simulink model "Lcontainer_sim"  (R2018b)
settings: Solver=ode1  StartTime=0.0  StopTime=600  FixedStep=0.1  RelTol=1e-3
libraries: neural x49, simulink x2
(part 2 of 2)

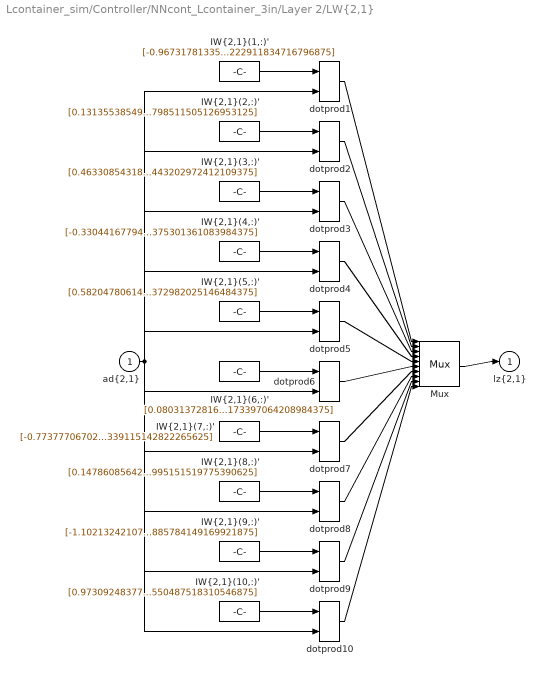
== system Lcontainer_sim/Controller/NNcont_Lcontainer_3in/Layer 2/LW{2,1} ==
  "ad{2,1}" : Inport  PortDimensions=10
      mask Display: e = 0.06;c1 = [120 230 180]/255;c2 = ([120 230 180]+0)/(256+128);c3 = ([120 230 180]+128)/(256+128);patch([0 1 1 0],[0 0 1 1],c1);patch([0 1 1 1-e 1-e 0+e],[0 0 1 1-e 0+e 0+e],c2);patch([0 0 1 1-e 0+e 0+e],[0 1 1 1-e 1-e 0+e],c3);plot([0 1 1 0 0],[0 0 1 1 0]);
  "IW{2,1}(1,:)'" : Constant  Value=[-0.9673178133559503510952026772429235279560089111328125;0.53839778171147634200366383083746768534183502197265625;-0.722317642025362971480717533268034458160400390625;0.8553552777126747219682556533371098339557647705078125;0.275878338813815293661946270731277763843536376953125;-0.02755546810020788328632335151269217021763324737548828125;0.82237984032601907369297578043187968432903289794921875;-0.2547472202517508943486745920381508767604827880859375;-0.61557536337765605960470338686718605458736419677734375;0.153664159931131638625600999148446135222911834716796875]
      mask Display: e = 0.06;c1 = [120 150 230]/255;c2 = ([120 150 230]+0)/383;c3 = ([120 150 230]+128)/383;patch([0 1 1 0],[0 0 1 1],c1);patch([0 1 1 1-e 1-e 0+e],[0 0 1 1-e 0+e 0+e],c2);patch([0 0 1 1-e 0+e 0+e],[0 1 1 1-e 1-e 0+e],c3);plot([0 1 1 0 0],[0 0 1 1 0]);disp('weights');
  "IW{2,1}(10,:)'" : Constant  Value=[0.97309248377746315750158601076691411435604095458984375;-0.845856659992735959718856975086964666843414306640625;0.0295346903368784718946216116819414310157299041748046875;-1.1110911960074727478087197596323676407337188720703125;0.3060928624502607942048371114651672542095184326171875;-0.026387217399169611564690995919590932317078113555908203125;-0.554579983764879269614311851910315454006195068359375;-0.7959887047101454893294203429832123219966888427734375;-0.53675247865637409905303911727969534695148468017578125;-0.30786197281541471948429489202680997550487518310546875]
      mask Display: e = 0.06;c1 = [120 150 230]/255;c2 = ([120 150 230]+0)/383;c3 = ([120 150 230]+128)/383;patch([0 1 1 0],[0 0 1 1],c1);patch([0 1 1 1-e 1-e 0+e],[0 0 1 1-e 0+e 0+e],c2);patch([0 0 1 1-e 0+e 0+e],[0 1 1 1-e 1-e 0+e],c3);plot([0 1 1 0 0],[0 0 1 1 0]);disp('weights');
  "IW{2,1}(2,:)'" : Constant  Value=[0.1313553854999522096935749004842364229261875152587890625;-0.79774829886561471337103057521744631230831146240234375;-0.286014502405725845601835999332251958549022674560546875;1.1879656245342637976847299796645529568195343017578125;-0.70701622775883998794910212382092140614986419677734375;0.1677083387146580395477002412008005194365978240966796875;-0.46969451886407587171134991876897402107715606689453125;-0.138127570352924611274403332572546787559986114501953125;-0.43525645097113885295669888364500366151332855224609375;0.050289888408718404211317221097488072700798511505126953125]
      mask Display: e = 0.06;c1 = [120 150 230]/255;c2 = ([120 150 230]+0)/383;c3 = ([120 150 230]+128)/383;patch([0 1 1 0],[0 0 1 1],c1);patch([0 1 1 1-e 1-e 0+e],[0 0 1 1-e 0+e 0+e],c2);patch([0 0 1 1-e 0+e 0+e],[0 1 1 1-e 1-e 0+e],c3);plot([0 1 1 0 0],[0 0 1 1 0]);disp('weights');
  "IW{2,1}(3,:)'" : Constant  Value=[0.463308543185886156923203316182480193674564361572265625;0.01474050328529204374750083417211499181576073169708251953125;0.5708458173938455448848117157467640936374664306640625;-0.36304390338556735695618726822431199252605438232421875;0.03802927902901009904468310196534730494022369384765625;0.8688905579410917123794888539123348891735076904296875;-0.368022670402931073585506283052382059395313262939453125;1.078571025995817223019912489689886569976806640625;-0.42042514591632340614779650422860868275165557861328125;0.449357619793621321235832510865293443202972412109375]
      mask Display: e = 0.06;c1 = [120 150 230]/255;c2 = ([120 150 230]+0)/383;c3 = ([120 150 230]+128)/383;patch([0 1 1 0],[0 0 1 1],c1);patch([0 1 1 1-e 1-e 0+e],[0 0 1 1-e 0+e 0+e],c2);patch([0 0 1 1-e 0+e 0+e],[0 1 1 1-e 1-e 0+e],c3);plot([0 1 1 0 0],[0 0 1 1 0]);disp('weights');
  "IW{2,1}(4,:)'" : Constant  Value=[-0.330441677946859357906106424707104451954364776611328125;0.9398932320279040908417300670407712459564208984375;0.024098708014007048927584975217541796155273914337158203125;0.4618698985408240531569390441291034221649169921875;-1.1397682984094237301775365267531014978885650634765625;0.860210379926586110599373569129966199398040771484375;-0.17513721026530471025495216963463462889194488525390625;-0.410569653732319128636163441115058958530426025390625;-0.5560344839229272029257344911457039415836334228515625;-0.308418252656767977182283857473521493375301361083984375]
      mask Display: e = 0.06;c1 = [120 150 230]/255;c2 = ([120 150 230]+0)/383;c3 = ([120 150 230]+128)/383;patch([0 1 1 0],[0 0 1 1],c1);patch([0 1 1 1-e 1-e 0+e],[0 0 1 1-e 0+e 0+e],c2);patch([0 0 1 1-e 0+e 0+e],[0 1 1 1-e 1-e 0+e],c3);plot([0 1 1 0 0],[0 0 1 1 0]);disp('weights');
  "IW{2,1}(5,:)'" : Constant  Value=[0.58204780614894213730536876028054393827915191650390625;0.6967907615499668860792326086084358394145965576171875;0.99667255359175188633713560193427838385105133056640625;-0.699431723040012887082639281288720667362213134765625;-0.46866769281885722886471512538264505565166473388671875;-0.140751847389412765298999374863342382013797760009765625;0.12716603274524984623639056735555641353130340576171875;0.62879100504427842821542071760632097721099853515625;0.18062992316508286183562859150697477161884307861328125;0.3404346384178766893313650143682025372982025146484375]
      mask Display: e = 0.06;c1 = [120 150 230]/255;c2 = ([120 150 230]+0)/383;c3 = ([120 150 230]+128)/383;patch([0 1 1 0],[0 0 1 1],c1);patch([0 1 1 1-e 1-e 0+e],[0 0 1 1-e 0+e 0+e],c2);patch([0 0 1 1-e 0+e 0+e],[0 1 1 1-e 1-e 0+e],c3);plot([0 1 1 0 0],[0 0 1 1 0]);disp('weights');
  "IW{2,1}(6,:)'" : Constant  Value=[0.08031372816249911228414504194006440229713916778564453125;-0.297973938059601428651745891329483129084110260009765625;0.64300070459735680916679712026962079107761383056640625;0.53040993310285677875270948788966052234172821044921875;-0.79049086677915136878169732881360687315464019775390625;0.0832509692935996803431208945767139084637165069580078125;0.718295773451751440319412722601555287837982177734375;0.2364318776000905175660449231145321391522884368896484375;-0.8074693176251519499686537528759799897670745849609375;-0.80866490504699528596432855920284055173397064208984375]
      mask Display: e = 0.06;c1 = [120 150 230]/255;c2 = ([120 150 230]+0)/383;c3 = ([120 150 230]+128)/383;patch([0 1 1 0],[0 0 1 1],c1);patch([0 1 1 1-e 1-e 0+e],[0 0 1 1-e 0+e 0+e],c2);patch([0 0 1 1-e 0+e 0+e],[0 1 1 1-e 1-e 0+e],c3);plot([0 1 1 0 0],[0 0 1 1 0]);disp('weights');
  "IW{2,1}(7,:)'" : Constant  Value=[-0.77377706702885273859493509007734246551990509033203125;0.376757424003904883846871598507277667522430419921875;-0.19997543976920895136828448812593705952167510986328125;0.70509502994817807586258595620165579020977020263671875;0.06363014764948270174382827235604054294526576995849609375;0.70247114849747216425157603225670754909515380859375;-0.57831088496463889381260514710447750985622406005859375;-0.2346865136461891709895866142687737010419368743896484375;0.312603908634070337679844442391186021268367767333984375;-0.91858990863328193743342353627667762339115142822265625]
      mask Display: e = 0.06;c1 = [120 150 230]/255;c2 = ([120 150 230]+0)/383;c3 = ([120 150 230]+128)/383;patch([0 1 1 0],[0 0 1 1],c1);patch([0 1 1 1-e 1-e 0+e],[0 0 1 1-e 0+e 0+e],c2);patch([0 0 1 1-e 0+e 0+e],[0 1 1 1-e 1-e 0+e],c3);plot([0 1 1 0 0],[0 0 1 1 0]);disp('weights');
  "IW{2,1}(8,:)'" : Constant  Value=[0.1478608564296591543207881613852805458009243011474609375;0.664531605347525644589268267736770212650299072265625;-0.441801587802395701043423059672932140529155731201171875;0.69565887282337224295503119719796814024448394775390625;0.00545381413161631113661886871568640344776213169097900390625;-0.92106408854380183992560660044546239078044891357421875;0.033361495389616628581830326538693043403327465057373046875;-0.79809310204494388063523047094349749386310577392578125;0.71885462226626295478837391783599741756916046142578125;-0.6699848944034219044851852231658995151519775390625]
      mask Display: e = 0.06;c1 = [120 150 230]/255;c2 = ([120 150 230]+0)/383;c3 = ([120 150 230]+128)/383;patch([0 1 1 0],[0 0 1 1],c1);patch([0 1 1 1-e 1-e 0+e],[0 0 1 1-e 0+e 0+e],c2);patch([0 0 1 1-e 0+e 0+e],[0 1 1 1-e 1-e 0+e],c3);plot([0 1 1 0 0],[0 0 1 1 0]);disp('weights');
  "IW{2,1}(9,:)'" : Constant  Value=[-1.102132421071642998100514887482859194278717041015625;-0.6682571900111622387186116611701436340808868408203125;0.292635550191234827810404794945497997105121612548828125;-0.2314539238324496983612021949738846160471439361572265625;0.57375985909356630454425385323702357709407806396484375;0.06759075797283618791677639592307968996465206146240234375;-0.52314955273553220838067545628291554749011993408203125;-0.2028998165833909295141523898564628325402736663818359375;0.66713933922251789088164741770015098154544830322265625;-0.460676733779915970057317053942824713885784149169921875]
      mask Display: e = 0.06;c1 = [120 150 230]/255;c2 = ([120 150 230]+0)/383;c3 = ([120 150 230]+128)/383;patch([0 1 1 0],[0 0 1 1],c1);patch([0 1 1 1-e 1-e 0+e],[0 0 1 1-e 0+e 0+e],c2);patch([0 0 1 1-e 0+e 0+e],[0 1 1 1-e 1-e 0+e],c3);plot([0 1 1 0 0],[0 0 1 1 0]);disp('weights');
  Mux : Mux  Inputs=10
      mask Display: e = 0.06;c1 = [120 150 230]/255;c2 = ([120 150 230]+0)/383;c3 = ([120 150 230]+128)/383;patch([0 1 1 0],[0 0 1 1],c1);patch([0 1 1 1-e 1-e 0+e],[0 0 1 1-e 0+e 0+e],c2);patch([0 0 1 1-e 0+e 0+e],[0 1 1 1-e 1-e 0+e],c3);plot([0 1 1 0 0],[0 0 1 1 0]);disp('Mux');
  dotprod{1..10} (10 alike) : neural/Weight Functions/dotprod
  "lz{2,1}" : Outport
      mask Display: e = 0.06;c1 = [120 230 180]/255;c2 = ([120 230 180]+0)/(256+128);c3 = ([120 230 180]+128)/(256+128);patch([0 1 1 0],[0 0 1 1],c1);patch([0 1 1 1-e 1-e 0+e],[0 0 1 1-e 0+e 0+e],c2);patch([0 0 1 1-e 0+e 0+e],[0 1 1 1-e 1-e 0+e],c3);plot([0 1 1 0 0],[0 0 1 1 0]);
  wires:
  Mux/1 -> "lz{2,1}"/1
  dotprod10/1 -> Mux/10
  "IW{2,1}(10,:)'"/1 -> dotprod10/1
  dotprod9/1 -> Mux/9
  "IW{2,1}(9,:)'"/1 -> dotprod9/1
  dotprod8/1 -> Mux/8
  "IW{2,1}(8,:)'"/1 -> dotprod8/1
  dotprod7/1 -> Mux/7
  "IW{2,1}(7,:)'"/1 -> dotprod7/1
  dotprod6/1 -> Mux/6
  "IW{2,1}(6,:)'"/1 -> dotprod6/1
  dotprod5/1 -> Mux/5
  "IW{2,1}(5,:)'"/1 -> dotprod5/1
  dotprod4/1 -> Mux/4
  "IW{2,1}(4,:)'"/1 -> dotprod4/1
  dotprod3/1 -> Mux/3
  "IW{2,1}(3,:)'"/1 -> dotprod3/1
  dotprod2/1 -> Mux/2
  "IW{2,1}(2,:)'"/1 -> dotprod2/1
  dotprod1/1 -> Mux/1
  "ad{2,1}"/1 -> dotprod10/2, dotprod9/2, dotprod8/2, dotprod7/2, dotprod6/2, dotprod5/2, dotprod4/2, dotprod3/2, dotprod2/2, dotprod1/2
  "IW{2,1}(1,:)'"/1 -> dotprod1/1

== system Lcontainer_sim/Controller/NNcont_Lcontainer_3in/Layer 3/Delays 1 ==
  "p{3}" : Inport  PortDimensions=10
      mask Display: e = 0.06;c1 = [120 230 180]/255;c2 = ([120 230 180]+0)/(256+128);c3 = ([120 230 180]+128)/(256+128);patch([0 1 1 0],[0 0 1 1],c1);patch([0 1 1 1-e 1-e 0+e],[0 0 1 1-e 0+e 0+e],c2);patch([0 0 1 1-e 0+e 0+e],[0 1 1 1-e 1-e 0+e],c3);plot([0 1 1 0 0],[0 0 1 1 0]);
  mux : Mux  Inputs=1
      mask Display: e = 0.06;c1 = [120 150 230]/255;c2 = ([120 150 230]+0)/383;c3 = ([120 150 230]+128)/383;patch([0 1 1 0],[0 0 1 1],c1);patch([0 1 1 1-e 1-e 0+e],[0 0 1 1-e 0+e 0+e],c2);patch([0 0 1 1-e 0+e 0+e],[0 1 1 1-e 1-e 0+e],c3);plot([0 1 1 0 0],[0 0 1 1 0]);disp('Mux')
  "pd{3,2}" : Outport
      mask Display: e = 0.06;c1 = [120 230 180]/255;c2 = ([120 230 180]+0)/(256+128);c3 = ([120 230 180]+128)/(256+128);patch([0 1 1 0],[0 0 1 1],c1);patch([0 1 1 1-e 1-e 0+e],[0 0 1 1-e 0+e 0+e],c2);patch([0 0 1 1-e 0+e 0+e],[0 1 1 1-e 1-e 0+e],c3);plot([0 1 1 0 0],[0 0 1 1 0]);
  wires:
  mux/1 -> "pd{3,2}"/1
  "p{3}"/1 -> mux/1

== system Lcontainer_sim/Controller/NNcont_Lcontainer_3in/Layer 3/LW{3,2} ==
  "ad{3,2}" : Inport  PortDimensions=10
      mask Display: e = 0.06;c1 = [120 230 180]/255;c2 = ([120 230 180]+0)/(256+128);c3 = ([120 230 180]+128)/(256+128);patch([0 1 1 0],[0 0 1 1],c1);patch([0 1 1 1-e 1-e 0+e],[0 0 1 1-e 0+e 0+e],c2);patch([0 0 1 1-e 0+e 0+e],[0 1 1 1-e 1-e 0+e],c3);plot([0 1 1 0 0],[0 0 1 1 0]);
  "IW{3,2}(1,:)'" : Constant  Value=[-0.73149029744197668900795861190999858081340789794921875;0;0;-0.84948708100111236518614532542414963245391845703125;0;-0.437042300450375176268380528199486434459686279296875;0;-0.66202787718184818999134222394786775112152099609375;0;1.1687904609959163249044422627775929868221282958984375]
      mask Display: e = 0.06;c1 = [120 150 230]/255;c2 = ([120 150 230]+0)/383;c3 = ([120 150 230]+128)/383;patch([0 1 1 0],[0 0 1 1],c1);patch([0 1 1 1-e 1-e 0+e],[0 0 1 1-e 0+e 0+e],c2);patch([0 0 1 1-e 0+e 0+e],[0 1 1 1-e 1-e 0+e],c3);plot([0 1 1 0 0],[0 0 1 1 0]);disp('weights');
  Mux : Mux  Inputs=1
      mask Display: e = 0.06;c1 = [120 150 230]/255;c2 = ([120 150 230]+0)/383;c3 = ([120 150 230]+128)/383;patch([0 1 1 0],[0 0 1 1],c1);patch([0 1 1 1-e 1-e 0+e],[0 0 1 1-e 0+e 0+e],c2);patch([0 0 1 1-e 0+e 0+e],[0 1 1 1-e 1-e 0+e],c3);plot([0 1 1 0 0],[0 0 1 1 0]);disp('Mux');
  dotprod1 : neural/Weight Functions/dotprod
  "lz{3,2}" : Outport
      mask Display: e = 0.06;c1 = [120 230 180]/255;c2 = ([120 230 180]+0)/(256+128);c3 = ([120 230 180]+128)/(256+128);patch([0 1 1 0],[0 0 1 1],c1);patch([0 1 1 1-e 1-e 0+e],[0 0 1 1-e 0+e 0+e],c2);patch([0 0 1 1-e 0+e 0+e],[0 1 1 1-e 1-e 0+e],c3);plot([0 1 1 0 0],[0 0 1 1 0]);
  wires:
  Mux/1 -> "lz{3,2}"/1
  dotprod1/1 -> Mux/1
  "ad{3,2}"/1 -> dotprod1/2
  "IW{3,2}(1,:)'"/1 -> dotprod1/1

== system Lcontainer_sim/Controller/controller_Lcontainer_3in/Layer 1/Delays 1 ==
  "p{1}" : Inport  PortDimensions=3
      mask Display: e = 0.06;c1 = [120 230 180]/255;c2 = ([120 230 180]+0)/(256+128);c3 = ([120 230 180]+128)/(256+128);patch([0 1 1 0],[0 0 1 1],c1);patch([0 1 1 1-e 1-e 0+e],[0 0 1 1-e 0+e 0+e],c2);patch([0 0 1 1-e 0+e 0+e],[0 1 1 1-e 1-e 0+e],c3);plot([0 1 1 0 0],[0 0 1 1 0]);
  mux : Mux  Inputs=1
      mask Display: e = 0.06;c1 = [120 150 230]/255;c2 = ([120 150 230]+0)/383;c3 = ([120 150 230]+128)/383;patch([0 1 1 0],[0 0 1 1],c1);patch([0 1 1 1-e 1-e 0+e],[0 0 1 1-e 0+e 0+e],c2);patch([0 0 1 1-e 0+e 0+e],[0 1 1 1-e 1-e 0+e],c3);plot([0 1 1 0 0],[0 0 1 1 0]);disp('Mux')
  "pd{1,1}" : Outport
      mask Display: e = 0.06;c1 = [120 230 180]/255;c2 = ([120 230 180]+0)/(256+128);c3 = ([120 230 180]+128)/(256+128);patch([0 1 1 0],[0 0 1 1],c1);patch([0 1 1 1-e 1-e 0+e],[0 0 1 1-e 0+e 0+e],c2);patch([0 0 1 1-e 0+e 0+e],[0 1 1 1-e 1-e 0+e],c3);plot([0 1 1 0 0],[0 0 1 1 0]);
  wires:
  mux/1 -> "pd{1,1}"/1
  "p{1}"/1 -> mux/1

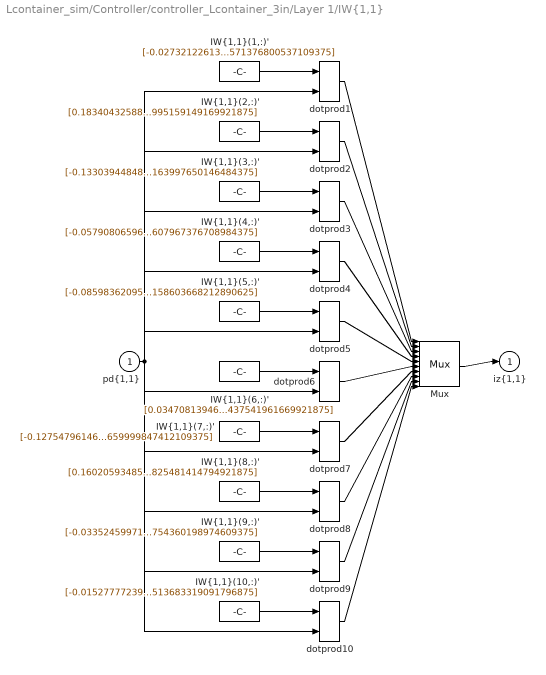
== system Lcontainer_sim/Controller/controller_Lcontainer_3in/Layer 1/IW{1,1} ==
  "pd{1,1}" : Inport  PortDimensions=3
      mask Display: e = 0.06;c1 = [120 230 180]/255;c2 = ([120 230 180]+0)/(256+128);c3 = ([120 230 180]+128)/(256+128);patch([0 1 1 0],[0 0 1 1],c1);patch([0 1 1 1-e 1-e 0+e],[0 0 1 1-e 0+e 0+e],c2);patch([0 0 1 1-e 0+e 0+e],[0 1 1 1-e 1-e 0+e],c3);plot([0 1 1 0 0],[0 0 1 1 0]);
  "IW{1,1}(1,:)'" : Constant  Value=[-0.0273212261328430149054380393636165536008775234222412109375;1.2466153438031797318075177827267907559871673583984375;-0.481779587181954516150739209479070268571376800537109375]
      mask Display: e = 0.06;c1 = [120 150 230]/255;c2 = ([120 150 230]+0)/383;c3 = ([120 150 230]+128)/383;patch([0 1 1 0],[0 0 1 1],c1);patch([0 1 1 1-e 1-e 0+e],[0 0 1 1-e 0+e 0+e],c2);patch([0 0 1 1-e 0+e 0+e],[0 1 1 1-e 1-e 0+e],c3);plot([0 1 1 0 0],[0 0 1 1 0]);disp('Weights');
  "IW{1,1}(10,:)'" : Constant  Value=[-0.0152777723937224697847714338649893761612474918365478515625;0.61986865608767971469461599554051645100116729736328125;-0.324049322408245632498591248804586939513683319091796875]
      mask Display: e = 0.06;c1 = [120 150 230]/255;c2 = ([120 150 230]+0)/383;c3 = ([120 150 230]+128)/383;patch([0 1 1 0],[0 0 1 1],c1);patch([0 1 1 1-e 1-e 0+e],[0 0 1 1-e 0+e 0+e],c2);patch([0 0 1 1-e 0+e 0+e],[0 1 1 1-e 1-e 0+e],c3);plot([0 1 1 0 0],[0 0 1 1 0]);disp('Weights');
  "IW{1,1}(2,:)'" : Constant  Value=[0.1834043258807954990263766603675321675837039947509765625;-7.5868248635884985020538806566037237644195556640625;3.854324903699683613211846022750250995159149169921875]
      mask Display: e = 0.06;c1 = [120 150 230]/255;c2 = ([120 150 230]+0)/383;c3 = ([120 150 230]+128)/383;patch([0 1 1 0],[0 0 1 1],c1);patch([0 1 1 1-e 1-e 0+e],[0 0 1 1-e 0+e 0+e],c2);patch([0 0 1 1-e 0+e 0+e],[0 1 1 1-e 1-e 0+e],c3);plot([0 1 1 0 0],[0 0 1 1 0]);disp('Weights');
  "IW{1,1}(3,:)'" : Constant  Value=[-0.1330394484899174167846780392210348509252071380615234375;5.1403328302688340301074276794679462909698486328125;-3.191619900639112383800011230050586163997650146484375]
      mask Display: e = 0.06;c1 = [120 150 230]/255;c2 = ([120 150 230]+0)/383;c3 = ([120 150 230]+128)/383;patch([0 1 1 0],[0 0 1 1],c1);patch([0 1 1 1-e 1-e 0+e],[0 0 1 1-e 0+e 0+e],c2);patch([0 0 1 1-e 0+e 0+e],[0 1 1 1-e 1-e 0+e],c3);plot([0 1 1 0 0],[0 0 1 1 0]);disp('Weights');
  "IW{1,1}(4,:)'" : Constant  Value=[-0.057908065963439024625980522387180826626718044281005859375;2.3372705025380877685847735847346484661102294921875;-1.2846422947148086191049287663190625607967376708984375]
      mask Display: e = 0.06;c1 = [120 150 230]/255;c2 = ([120 150 230]+0)/383;c3 = ([120 150 230]+128)/383;patch([0 1 1 0],[0 0 1 1],c1);patch([0 1 1 1-e 1-e 0+e],[0 0 1 1-e 0+e 0+e],c2);patch([0 0 1 1-e 0+e 0+e],[0 1 1 1-e 1-e 0+e],c3);plot([0 1 1 0 0],[0 0 1 1 0]);disp('Weights');
  "IW{1,1}(5,:)'" : Constant  Value=[-0.08598362095952950812094428556520142592489719390869140625;3.591099600093372146147885359823703765869140625;-1.7613597454396379138330530622624792158603668212890625]
      mask Display: e = 0.06;c1 = [120 150 230]/255;c2 = ([120 150 230]+0)/383;c3 = ([120 150 230]+128)/383;patch([0 1 1 0],[0 0 1 1],c1);patch([0 1 1 1-e 1-e 0+e],[0 0 1 1-e 0+e 0+e],c2);patch([0 0 1 1-e 0+e 0+e],[0 1 1 1-e 1-e 0+e],c3);plot([0 1 1 0 0],[0 0 1 1 0]);disp('Weights');
  "IW{1,1}(6,:)'" : Constant  Value=[0.03470813946434479768665681831407709978520870208740234375;-1.328396893026822400685205138870514929294586181640625;0.82331844604563719780543351589585654437541961669921875]
      mask Display: e = 0.06;c1 = [120 150 230]/255;c2 = ([120 150 230]+0)/383;c3 = ([120 150 230]+128)/383;patch([0 1 1 0],[0 0 1 1],c1);patch([0 1 1 1-e 1-e 0+e],[0 0 1 1-e 0+e 0+e],c2);patch([0 0 1 1-e 0+e 0+e],[0 1 1 1-e 1-e 0+e],c3);plot([0 1 1 0 0],[0 0 1 1 0]);disp('Weights');
  "IW{1,1}(7,:)'" : Constant  Value=[-0.1275479614629743407849815639565349556505680084228515625;5.11845521089742927500765290460549294948577880859375;-2.879990022121622583739508627331815659999847412109375]
      mask Display: e = 0.06;c1 = [120 150 230]/255;c2 = ([120 150 230]+0)/383;c3 = ([120 150 230]+128)/383;patch([0 1 1 0],[0 0 1 1],c1);patch([0 1 1 1-e 1-e 0+e],[0 0 1 1-e 0+e 0+e],c2);patch([0 0 1 1-e 0+e 0+e],[0 1 1 1-e 1-e 0+e],c3);plot([0 1 1 0 0],[0 0 1 1 0]);disp('Weights');
  "IW{1,1}(8,:)'" : Constant  Value=[0.1602059348583863840342900175528484396636486053466796875;-6.42497549565498804469143578899092972278594970703125;3.579989609625108482049427038873545825481414794921875]
      mask Display: e = 0.06;c1 = [120 150 230]/255;c2 = ([120 150 230]+0)/383;c3 = ([120 150 230]+128)/383;patch([0 1 1 0],[0 0 1 1],c1);patch([0 1 1 1-e 1-e 0+e],[0 0 1 1-e 0+e 0+e],c2);patch([0 0 1 1-e 0+e 0+e],[0 1 1 1-e 1-e 0+e],c3);plot([0 1 1 0 0],[0 0 1 1 0]);disp('Weights');
  "IW{1,1}(9,:)'" : Constant  Value=[-0.03352459971025410767619945318074314855039119720458984375;1.3788408238072407119290119226207025349140167236328125;-0.7331232805546823438902492853230796754360198974609375]
      mask Display: e = 0.06;c1 = [120 150 230]/255;c2 = ([120 150 230]+0)/383;c3 = ([120 150 230]+128)/383;patch([0 1 1 0],[0 0 1 1],c1);patch([0 1 1 1-e 1-e 0+e],[0 0 1 1-e 0+e 0+e],c2);patch([0 0 1 1-e 0+e 0+e],[0 1 1 1-e 1-e 0+e],c3);plot([0 1 1 0 0],[0 0 1 1 0]);disp('Weights');
  Mux : Mux  Inputs=10
      mask Display: e = 0.06;c1 = [120 150 230]/255;c2 = ([120 150 230]+0)/383;c3 = ([120 150 230]+128)/383;patch([0 1 1 0],[0 0 1 1],c1);patch([0 1 1 1-e 1-e 0+e],[0 0 1 1-e 0+e 0+e],c2);patch([0 0 1 1-e 0+e 0+e],[0 1 1 1-e 1-e 0+e],c3);plot([0 1 1 0 0],[0 0 1 1 0]);disp('Mux');
  dotprod{1..10} (10 alike) : neural/Weight Functions/dotprod
  "iz{1,1}" : Outport
      mask Display: e = 0.06;c1 = [120 230 180]/255;c2 = ([120 230 180]+0)/(256+128);c3 = ([120 230 180]+128)/(256+128);patch([0 1 1 0],[0 0 1 1],c1);patch([0 1 1 1-e 1-e 0+e],[0 0 1 1-e 0+e 0+e],c2);patch([0 0 1 1-e 0+e 0+e],[0 1 1 1-e 1-e 0+e],c3);plot([0 1 1 0 0],[0 0 1 1 0]);
  wires:
  Mux/1 -> "iz{1,1}"/1
  dotprod10/1 -> Mux/10
  "IW{1,1}(10,:)'"/1 -> dotprod10/1
  dotprod9/1 -> Mux/9
  "IW{1,1}(9,:)'"/1 -> dotprod9/1
  dotprod8/1 -> Mux/8
  "IW{1,1}(8,:)'"/1 -> dotprod8/1
  dotprod7/1 -> Mux/7
  "IW{1,1}(7,:)'"/1 -> dotprod7/1
  dotprod6/1 -> Mux/6
  "IW{1,1}(6,:)'"/1 -> dotprod6/1
  dotprod5/1 -> Mux/5
  "IW{1,1}(5,:)'"/1 -> dotprod5/1
  dotprod4/1 -> Mux/4
  "IW{1,1}(4,:)'"/1 -> dotprod4/1
  dotprod3/1 -> Mux/3
  "IW{1,1}(3,:)'"/1 -> dotprod3/1
  dotprod2/1 -> Mux/2
  "IW{1,1}(2,:)'"/1 -> dotprod2/1
  dotprod1/1 -> Mux/1
  "pd{1,1}"/1 -> dotprod10/2, dotprod9/2, dotprod8/2, dotprod7/2, dotprod6/2, dotprod5/2, dotprod4/2, dotprod3/2, dotprod2/2, dotprod1/2
  "IW{1,1}(1,:)'"/1 -> dotprod1/1

== system Lcontainer_sim/Controller/controller_Lcontainer_3in/Layer 2/Delays 1 ==
  "p{2}" : Inport  PortDimensions=10
      mask Display: e = 0.06;c1 = [120 230 180]/255;c2 = ([120 230 180]+0)/(256+128);c3 = ([120 230 180]+128)/(256+128);patch([0 1 1 0],[0 0 1 1],c1);patch([0 1 1 1-e 1-e 0+e],[0 0 1 1-e 0+e 0+e],c2);patch([0 0 1 1-e 0+e 0+e],[0 1 1 1-e 1-e 0+e],c3);plot([0 1 1 0 0],[0 0 1 1 0]);
  mux : Mux  Inputs=1
      mask Display: e = 0.06;c1 = [120 150 230]/255;c2 = ([120 150 230]+0)/383;c3 = ([120 150 230]+128)/383;patch([0 1 1 0],[0 0 1 1],c1);patch([0 1 1 1-e 1-e 0+e],[0 0 1 1-e 0+e 0+e],c2);patch([0 0 1 1-e 0+e 0+e],[0 1 1 1-e 1-e 0+e],c3);plot([0 1 1 0 0],[0 0 1 1 0]);disp('Mux')
  "pd{2,1}" : Outport
      mask Display: e = 0.06;c1 = [120 230 180]/255;c2 = ([120 230 180]+0)/(256+128);c3 = ([120 230 180]+128)/(256+128);patch([0 1 1 0],[0 0 1 1],c1);patch([0 1 1 1-e 1-e 0+e],[0 0 1 1-e 0+e 0+e],c2);patch([0 0 1 1-e 0+e 0+e],[0 1 1 1-e 1-e 0+e],c3);plot([0 1 1 0 0],[0 0 1 1 0]);
  wires:
  mux/1 -> "pd{2,1}"/1
  "p{2}"/1 -> mux/1

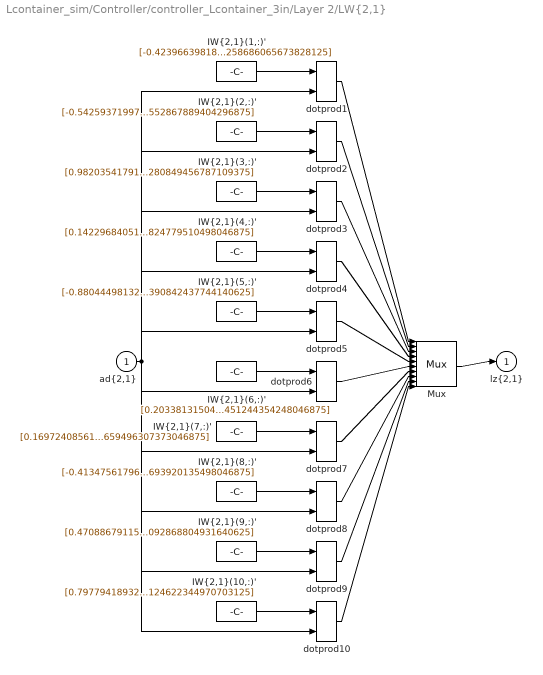
== system Lcontainer_sim/Controller/controller_Lcontainer_3in/Layer 2/LW{2,1} ==
  "ad{2,1}" : Inport  PortDimensions=10
      mask Display: e = 0.06;c1 = [120 230 180]/255;c2 = ([120 230 180]+0)/(256+128);c3 = ([120 230 180]+128)/(256+128);patch([0 1 1 0],[0 0 1 1],c1);patch([0 1 1 1-e 1-e 0+e],[0 0 1 1-e 0+e 0+e],c2);patch([0 0 1 1-e 0+e 0+e],[0 1 1 1-e 1-e 0+e],c3);plot([0 1 1 0 0],[0 0 1 1 0]);
  "IW{2,1}(1,:)'" : Constant  Value=[-0.423966398182069992284226600531837902963161468505859375;0.1997697189681837404151565351639874279499053955078125;0.85590666130776960063286651347880251705646514892578125;-0.202777735704410322359336760200676508247852325439453125;-0.607550791274205526093510343343950808048248291015625;0.183622508565573772099099869592464528977870941162109375;0.79342161690488499647955222826567478477954864501953125;-0.89935758921551312017328427828033454716205596923828125;0.5122530417571835581469485987327061593532562255859375;-0.20445057074798445029273352702148258686065673828125]
      mask Display: e = 0.06;c1 = [120 150 230]/255;c2 = ([120 150 230]+0)/383;c3 = ([120 150 230]+128)/383;patch([0 1 1 0],[0 0 1 1],c1);patch([0 1 1 1-e 1-e 0+e],[0 0 1 1-e 0+e 0+e],c2);patch([0 0 1 1-e 0+e 0+e],[0 1 1 1-e 1-e 0+e],c3);plot([0 1 1 0 0],[0 0 1 1 0]);disp('weights');
  "IW{2,1}(10,:)'" : Constant  Value=[0.79779418932987178347815415691002272069454193115234375;-1.16852019869485257430596902850084006786346435546875;0.11763801914301764972581310075838700868189334869384765625;0.2632036963965915798979722239891998469829559326171875;0.512491591075669550292559506488032639026641845703125;-0.482191199197833431089321720719453878700733184814453125;-0.00217976017672764747767910620268594357185065746307373046875;-0.525446018699392336515074930503033101558685302734375;-0.376526314807938133899511967683793045580387115478515625;0.32418991241792494140128155777347274124622344970703125]
      mask Display: e = 0.06;c1 = [120 150 230]/255;c2 = ([120 150 230]+0)/383;c3 = ([120 150 230]+128)/383;patch([0 1 1 0],[0 0 1 1],c1);patch([0 1 1 1-e 1-e 0+e],[0 0 1 1-e 0+e 0+e],c2);patch([0 0 1 1-e 0+e 0+e],[0 1 1 1-e 1-e 0+e],c3);plot([0 1 1 0 0],[0 0 1 1 0]);disp('weights');
  "IW{2,1}(2,:)'" : Constant  Value=[-0.54259371997224914441204646209371276199817657470703125;-0.64121626875647674825842159407329745590686798095703125;-0.54281828243952745527423076055129058659076690673828125;0.336391144536653474705900634944555349647998809814453125;0.312083482800655787059440626762807369232177734375;0.47754096539186041692204298669821582734584808349609375;0.64305653924021954903622599886148236691951751708984375;-0.535702354310083617150439749821089208126068115234375;0.736418180908254615957275746040977537631988525390625;0.64943366741279706655376458002137951552867889404296875]
      mask Display: e = 0.06;c1 = [120 150 230]/255;c2 = ([120 150 230]+0)/383;c3 = ([120 150 230]+128)/383;patch([0 1 1 0],[0 0 1 1],c1);patch([0 1 1 1-e 1-e 0+e],[0 0 1 1-e 0+e 0+e],c2);patch([0 0 1 1-e 0+e 0+e],[0 1 1 1-e 1-e 0+e],c3);plot([0 1 1 0 0],[0 0 1 1 0]);disp('weights');
  "IW{2,1}(3,:)'" : Constant  Value=[0.982035417912900499004535959102213382720947265625;-0.61498741185016003729657541043707169592380523681640625;0.66103506758305130563968532442231662571430206298828125;0.6217750021461105891518172938958741724491119384765625;0.10538250909773061447793907063896767795085906982421875;0.672556023768890565150968541274778544902801513671875;0.043514636978958014246199326180430944077670574188232421875;-0.101087211405337884517763313851901330053806304931640625;0.6043592353773326042443159167305566370487213134765625;-0.1824773230614170349550562377771711908280849456787109375]
      mask Display: e = 0.06;c1 = [120 150 230]/255;c2 = ([120 150 230]+0)/383;c3 = ([120 150 230]+128)/383;patch([0 1 1 0],[0 0 1 1],c1);patch([0 1 1 1-e 1-e 0+e],[0 0 1 1-e 0+e 0+e],c2);patch([0 0 1 1-e 0+e 0+e],[0 1 1 1-e 1-e 0+e],c3);plot([0 1 1 0 0],[0 0 1 1 0]);disp('weights');
  "IW{2,1}(4,:)'" : Constant  Value=[0.1422968405120259571816632160334847867488861083984375;0.58485482274428779447816850733943283557891845703125;-0.672007094924957915083041370962746441364288330078125;0.2179054462877716147328754914269666187465190887451171875;0.32458259693467217399387436671531759202480316162109375;-0.7914523210687516296957255690358579158782958984375;0.0184987806185031473937829815668010269291698932647705078125;-0.407518869106559489257080031165969558060169219970703125;0.416250077105763838236640594914206303656101226806640625;1.0833199825327166632149555880459956824779510498046875]
      mask Display: e = 0.06;c1 = [120 150 230]/255;c2 = ([120 150 230]+0)/383;c3 = ([120 150 230]+128)/383;patch([0 1 1 0],[0 0 1 1],c1);patch([0 1 1 1-e 1-e 0+e],[0 0 1 1-e 0+e 0+e],c2);patch([0 0 1 1-e 0+e 0+e],[0 1 1 1-e 1-e 0+e],c3);plot([0 1 1 0 0],[0 0 1 1 0]);disp('weights');
  "IW{2,1}(5,:)'" : Constant  Value=[-0.8804449813212205100398932700045406818389892578125;0.285521360360928955213211111185955815017223358154296875;0.254521023578359317784958193442435003817081451416015625;0.138055486337296084986547839434933848679065704345703125;-0.71805618068881249538293332079774700105190277099609375;0.68117534526491396729142024923930875957012176513671875;0.94044458754698201374822019715793430805206298828125;-0.3472788706421832127801962997182272374629974365234375;-0.04229827980680260501866740696641500107944011688232421875;0.43759490835867398406122674714424647390842437744140625]
      mask Display: e = 0.06;c1 = [120 150 230]/255;c2 = ([120 150 230]+0)/383;c3 = ([120 150 230]+128)/383;patch([0 1 1 0],[0 0 1 1],c1);patch([0 1 1 1-e 1-e 0+e],[0 0 1 1-e 0+e 0+e],c2);patch([0 0 1 1-e 0+e 0+e],[0 1 1 1-e 1-e 0+e],c3);plot([0 1 1 0 0],[0 0 1 1 0]);disp('weights');
  "IW{2,1}(6,:)'" : Constant  Value=[0.2033813150496447674786537618274451233446598052978515625;0.40429455771327360569245001897797919809818267822265625;-1.0287344923148815656332999424193985760211944580078125;-0.40695762899609178031568035294185392558574676513671875;-0.0994421458463171925590273758643888868391513824462890625;0.911690811968453029834336120984517037868499755859375;-0.25652903115582359472313100923202000558376312255859375;0.265410065888411372814204014503047801554203033447265625;0.1729178743478333168948068987447186373174190521240234375;-0.85381333894444277898827522221836261451244354248046875]
      mask Display: e = 0.06;c1 = [120 150 230]/255;c2 = ([120 150 230]+0)/383;c3 = ([120 150 230]+128)/383;patch([0 1 1 0],[0 0 1 1],c1);patch([0 1 1 1-e 1-e 0+e],[0 0 1 1-e 0+e 0+e],c2);patch([0 0 1 1-e 0+e 0+e],[0 1 1 1-e 1-e 0+e],c3);plot([0 1 1 0 0],[0 0 1 1 0]);disp('weights');
  "IW{2,1}(7,:)'" : Constant  Value=[0.1697240856179695056571432587588788010179996490478515625;0.6402350580861078110928019668790511786937713623046875;0.63996660172811548061844177937018685042858123779296875;0.2303929432914660069275925025067408569157123565673828125;0.81480844173445721168036470771767199039459228515625;-0.61290851319237449335020073704072274267673492431640625;-0.5631799256368668071814909126260317862033843994140625;-0.11949842718370586036602531976313912309706211090087890625;-0.254425894470766744692724614651524461805820465087890625;-0.87758243051585960170513089906307868659496307373046875]
      mask Display: e = 0.06;c1 = [120 150 230]/255;c2 = ([120 150 230]+0)/383;c3 = ([120 150 230]+128)/383;patch([0 1 1 0],[0 0 1 1],c1);patch([0 1 1 1-e 1-e 0+e],[0 0 1 1-e 0+e 0+e],c2);patch([0 0 1 1-e 0+e 0+e],[0 1 1 1-e 1-e 0+e],c3);plot([0 1 1 0 0],[0 0 1 1 0]);disp('weights');
  "IW{2,1}(8,:)'" : Constant  Value=[-0.413475617962977548547343076279503293335437774658203125;-0.59124449486275343357277733957744203507900238037109375;-0.673959056190555738652392392395995557308197021484375;0.416377344789815861947346320448559708893299102783203125;-0.69098558253785002936098180725821293890476226806640625;0.2144611510258989939270435343132703565061092376708984375;-0.27744967429855404983385369632742367684841156005859375;0.497885566970060755576099609243101440370082855224609375;0.060295821064150136037174121383941383101046085357666015625;-1.0518122498883168969285861749085597693920135498046875]
      mask Display: e = 0.06;c1 = [120 150 230]/255;c2 = ([120 150 230]+0)/383;c3 = ([120 150 230]+128)/383;patch([0 1 1 0],[0 0 1 1],c1);patch([0 1 1 1-e 1-e 0+e],[0 0 1 1-e 0+e 0+e],c2);patch([0 0 1 1-e 0+e 0+e],[0 1 1 1-e 1-e 0+e],c3);plot([0 1 1 0 0],[0 0 1 1 0]);disp('weights');
  "IW{2,1}(9,:)'" : Constant  Value=[0.470886791152280992367451517566223628818988800048828125;-0.9797622520185857997176981371012516319751739501953125;0.87644042460278914763449620295432396233081817626953125;0.297291861750680175280336925425217486917972564697265625;0.73276277502347764158940890411031432449817657470703125;-0.51191327758836557837440750517998822033405303955078125;0.1815559821563396403210077778567210771143436431884765625;0.27399010004052115618833340704441070556640625;-0.36868002480531159026355680907727219164371490478515625;-0.166039942343781776745714751086779870092868804931640625]
      mask Display: e = 0.06;c1 = [120 150 230]/255;c2 = ([120 150 230]+0)/383;c3 = ([120 150 230]+128)/383;patch([0 1 1 0],[0 0 1 1],c1);patch([0 1 1 1-e 1-e 0+e],[0 0 1 1-e 0+e 0+e],c2);patch([0 0 1 1-e 0+e 0+e],[0 1 1 1-e 1-e 0+e],c3);plot([0 1 1 0 0],[0 0 1 1 0]);disp('weights');
  Mux : Mux  Inputs=10
      mask Display: e = 0.06;c1 = [120 150 230]/255;c2 = ([120 150 230]+0)/383;c3 = ([120 150 230]+128)/383;patch([0 1 1 0],[0 0 1 1],c1);patch([0 1 1 1-e 1-e 0+e],[0 0 1 1-e 0+e 0+e],c2);patch([0 0 1 1-e 0+e 0+e],[0 1 1 1-e 1-e 0+e],c3);plot([0 1 1 0 0],[0 0 1 1 0]);disp('Mux');
  dotprod{1..10} (10 alike) : neural/Weight Functions/dotprod
  "lz{2,1}" : Outport
      mask Display: e = 0.06;c1 = [120 230 180]/255;c2 = ([120 230 180]+0)/(256+128);c3 = ([120 230 180]+128)/(256+128);patch([0 1 1 0],[0 0 1 1],c1);patch([0 1 1 1-e 1-e 0+e],[0 0 1 1-e 0+e 0+e],c2);patch([0 0 1 1-e 0+e 0+e],[0 1 1 1-e 1-e 0+e],c3);plot([0 1 1 0 0],[0 0 1 1 0]);
  wires:
  Mux/1 -> "lz{2,1}"/1
  dotprod10/1 -> Mux/10
  "IW{2,1}(10,:)'"/1 -> dotprod10/1
  dotprod9/1 -> Mux/9
  "IW{2,1}(9,:)'"/1 -> dotprod9/1
  dotprod8/1 -> Mux/8
  "IW{2,1}(8,:)'"/1 -> dotprod8/1
  dotprod7/1 -> Mux/7
  "IW{2,1}(7,:)'"/1 -> dotprod7/1
  dotprod6/1 -> Mux/6
  "IW{2,1}(6,:)'"/1 -> dotprod6/1
  dotprod5/1 -> Mux/5
  "IW{2,1}(5,:)'"/1 -> dotprod5/1
  dotprod4/1 -> Mux/4
  "IW{2,1}(4,:)'"/1 -> dotprod4/1
  dotprod3/1 -> Mux/3
  "IW{2,1}(3,:)'"/1 -> dotprod3/1
  dotprod2/1 -> Mux/2
  "IW{2,1}(2,:)'"/1 -> dotprod2/1
  dotprod1/1 -> Mux/1
  "ad{2,1}"/1 -> dotprod10/2, dotprod9/2, dotprod8/2, dotprod7/2, dotprod6/2, dotprod5/2, dotprod4/2, dotprod3/2, dotprod2/2, dotprod1/2
  "IW{2,1}(1,:)'"/1 -> dotprod1/1

== system Lcontainer_sim/Controller/controller_Lcontainer_3in/Layer 3/Delays 1 ==
  "p{3}" : Inport  PortDimensions=10
      mask Display: e = 0.06;c1 = [120 230 180]/255;c2 = ([120 230 180]+0)/(256+128);c3 = ([120 230 180]+128)/(256+128);patch([0 1 1 0],[0 0 1 1],c1);patch([0 1 1 1-e 1-e 0+e],[0 0 1 1-e 0+e 0+e],c2);patch([0 0 1 1-e 0+e 0+e],[0 1 1 1-e 1-e 0+e],c3);plot([0 1 1 0 0],[0 0 1 1 0]);
  mux : Mux  Inputs=1
      mask Display: e = 0.06;c1 = [120 150 230]/255;c2 = ([120 150 230]+0)/383;c3 = ([120 150 230]+128)/383;patch([0 1 1 0],[0 0 1 1],c1);patch([0 1 1 1-e 1-e 0+e],[0 0 1 1-e 0+e 0+e],c2);patch([0 0 1 1-e 0+e 0+e],[0 1 1 1-e 1-e 0+e],c3);plot([0 1 1 0 0],[0 0 1 1 0]);disp('Mux')
  "pd{3,2}" : Outport
      mask Display: e = 0.06;c1 = [120 230 180]/255;c2 = ([120 230 180]+0)/(256+128);c3 = ([120 230 180]+128)/(256+128);patch([0 1 1 0],[0 0 1 1],c1);patch([0 1 1 1-e 1-e 0+e],[0 0 1 1-e 0+e 0+e],c2);patch([0 0 1 1-e 0+e 0+e],[0 1 1 1-e 1-e 0+e],c3);plot([0 1 1 0 0],[0 0 1 1 0]);
  wires:
  mux/1 -> "pd{3,2}"/1
  "p{3}"/1 -> mux/1

== system Lcontainer_sim/Controller/controller_Lcontainer_3in/Layer 3/LW{3,2} ==
  "ad{3,2}" : Inport  PortDimensions=10
      mask Display: e = 0.06;c1 = [120 230 180]/255;c2 = ([120 230 180]+0)/(256+128);c3 = ([120 230 180]+128)/(256+128);patch([0 1 1 0],[0 0 1 1],c1);patch([0 1 1 1-e 1-e 0+e],[0 0 1 1-e 0+e 0+e],c2);patch([0 0 1 1-e 0+e 0+e],[0 1 1 1-e 1-e 0+e],c3);plot([0 1 1 0 0],[0 0 1 1 0]);
  "IW{3,2}(1,:)'" : Constant  Value=[-0.211062714102781157077259877041797153651714324951171875;0.1352041004300032767115880005803774110972881317138671875;-0.1976330856853815431950494030388654209673404693603515625;0;-0.2426357395715020570658992937751463614404201507568359375;0.05406884033851465376496747694545774720609188079833984375;0.045055404316779699980255458058309159241616725921630859375;0;-0.00664628160743902830775997614409789093770086765289306640625;0.0707593028954656977358439462477690540254116058349609375]
      mask Display: e = 0.06;c1 = [120 150 230]/255;c2 = ([120 150 230]+0)/383;c3 = ([120 150 230]+128)/383;patch([0 1 1 0],[0 0 1 1],c1);patch([0 1 1 1-e 1-e 0+e],[0 0 1 1-e 0+e 0+e],c2);patch([0 0 1 1-e 0+e 0+e],[0 1 1 1-e 1-e 0+e],c3);plot([0 1 1 0 0],[0 0 1 1 0]);disp('weights');
  Mux : Mux  Inputs=1
      mask Display: e = 0.06;c1 = [120 150 230]/255;c2 = ([120 150 230]+0)/383;c3 = ([120 150 230]+128)/383;patch([0 1 1 0],[0 0 1 1],c1);patch([0 1 1 1-e 1-e 0+e],[0 0 1 1-e 0+e 0+e],c2);patch([0 0 1 1-e 0+e 0+e],[0 1 1 1-e 1-e 0+e],c3);plot([0 1 1 0 0],[0 0 1 1 0]);disp('Mux');
  dotprod1 : neural/Weight Functions/dotprod
  "lz{3,2}" : Outport
      mask Display: e = 0.06;c1 = [120 230 180]/255;c2 = ([120 230 180]+0)/(256+128);c3 = ([120 230 180]+128)/(256+128);patch([0 1 1 0],[0 0 1 1],c1);patch([0 1 1 1-e 1-e 0+e],[0 0 1 1-e 0+e 0+e],c2);patch([0 0 1 1-e 0+e 0+e],[0 1 1 1-e 1-e 0+e],c3);plot([0 1 1 0 0],[0 0 1 1 0]);
  wires:
  Mux/1 -> "lz{3,2}"/1
  dotprod1/1 -> Mux/1
  "ad{3,2}"/1 -> dotprod1/2
  "IW{3,2}(1,:)'"/1 -> dotprod1/1

== matlab function Lcontainer_sim/MATLAB Function1 ==
  data: xdot input; xnext output; x input; h input
function xnext = euler2(xdot,x,h)
% EULER2  Integrate a system of ordinary differential equations using 
%	  Euler's 2nd-order method.
%
% xnext = euler2(xdot,x,h)
%
% xdot  - dx/dt(k) = f(x(k)
% x     - x(k)
% xnext - x(k+1)
% h     - step size
%
% Author:   Thor I. Fossen
% Date:     14th June 2001
% Revisions: 

xnext = x + h*xdot;

== matlab function Lcontainer_sim/LContainer plant ==
  data: x input; xdot output; ui input
function xdot = Lcontainer(x,ui)
% [xdot,U] = Lcontainer(x,ui,U0) returns the speed U in m/s (optionally) and the 
% time derivative of the state vector: x = [ u v r x y psi p phi delta ]'  using the
% the LINEARIZED model corresponding to the nonlinear model container.m. 
%
% u     = surge velocity          (m/s)
% v     = sway velocity           (m/s)
% r     = yaw velocity            (rad/s)
% x     = position in x-direction (m)
% y     = position in y-direction (m)
% psi   = yaw angle               (rad)
% p     = roll velocity           (rad/s)
% phi   = roll angle              (rad)
% delta = actual rudder angle     (rad)
%
% The inputs are :
%
% Uo     = service speed (optinally. Default speed U0 = 7 m/s
% ui     = commanded rudder angle   (rad)
%
% Reference:  Son og Nomoto (1982). On the Coupled Motion of Steering and 
%             Rolling of a High Speed Container Ship, Naval Architect of Ocean Engineering,
%             20: 73-83. From J.S.N.A. , Japan, Vol. 150, 1981.
% 
% Author:    Thor I. Fossen
% Date:      23rd July 2001
% Revisions: 

% Check of input and state dimensions
if (length(x) ~= 9),error('x-vector must have dimension 9 !');end

% Check of service speed
%if nargin==2, U0=7.0; end
U0 = 7.0;
%if U0 <=0,error('The ship must have speed greater than zero');end

% Normalization variables
rho = 1025;                 % water density (kg/m^3)
L = 175;                    % length of ship (m)
U = sqrt(U0^2 + x(2)^2);    % ship speed (m/s)

% rudder limitations
delta_max  = 10;             % max rudder angle (deg)
Ddelta_max = 5;              % max rudder rate (deg/s)

% States and inputs
delta_c = ui(1); 

v = x(2);     y = x(5);
r = x(3);   psi = x(6);
p = x(7);   phi = x(8);
nu    = [v r p]';   
eta   = [y psi phi]';
delta = x(9);    
 
% Linear model using nondimensional matrices and states with dimension (see Fossen 2002): 
% TM'inv(T) dv/dt + (U/L) TN'inv(T) v + (U/L)^2 TG'inv(T) eta = (U^2/L) T b' delta

T    = diag([ 1 1/L 1/L]);
Tinv = diag([ 1 L L ]);

M = [ 0.01497    0.0003525     -0.0002205       
      0.0003525  0.000875       0        
     -0.0002205  0              0.0000210 ];

N = [ 0.012035   0.00522    0   
      0.0038436  0.00243   -0.000213   
     -0.000314   0.0000692  0.0000075  ];

G = [ 0 0 0.0000704  
      0 0 0.0001468
      0 0 0.0004966 ];

b = [-0.002578 0.00126  0.0000855 ]';

% Rudder saturation and dynamics
if abs(delta_c) >= delta_max*pi/180,
   delta_c = sign(delta_c)*delta_max*pi/180;
end

delta_dot = delta_c - delta;
if abs(delta_dot) >= Ddelta_max*pi/180,
   delta_dot = sign(delta_dot)*Ddelta_max*pi/180;
end

% TM'inv(T) dv/dt + (U/L) TN'inv(T) v + (U/L)^2 TG'inv(T) eta = (U^2/L) T b' delta
nudot = inv(T*M*Tinv)*((U^2/L)*T*b*delta-(U/L)*T*N*Tinv*nu-(U/L)^2*T*G*Tinv*eta );

% Dimensional state derivatives xdot = [ u v r x y psi p phi delta ]'
xdot =[  0
         nudot(1)
         nudot(2)
         cos(psi)*U0-sin(psi)*cos(phi)*v
         sin(psi)*U0+cos(psi)*cos(phi)*v
         cos(phi)*r               
         nudot(3)
         p
         delta_dot                ];
